simulink model "ETMX"  (R2017b)
settings: Solver=VariableStepAuto  StartTime=0.0  StopTime=10.0  RelTol=1e-3
undefined symbols (not defined in the file): sys1
settings Model: Creator=ayaka  LastModifiedBy=ayaka

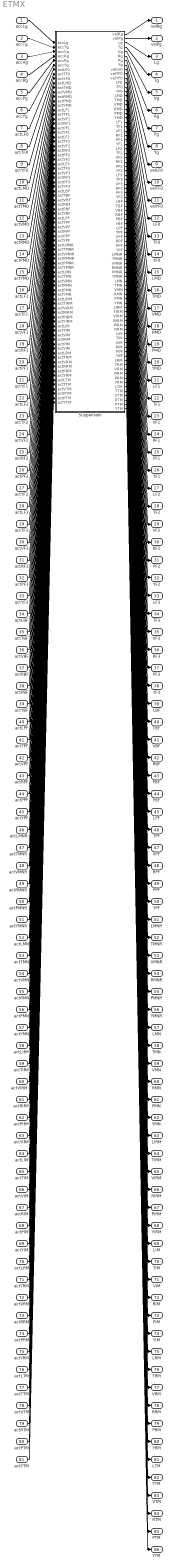
== system ETMX ==
  accLg : Inport
  accTg : Inport  Port=2
  accVg : Inport  Port=3
  accRg : Inport  Port=4
  accPg : Inport  Port=5
  accYg : Inport  Port=6
  actLF0 : Inport  Port=7
  actTF0 : Inport  Port=8
  actYF0 : Inport  Port=9
  actLMD : Inport  Port=10
  actTMD : Inport  Port=11
  actVMD : Inport  Port=12
  actRMD : Inport  Port=13
  actPMD : Inport  Port=14
  actYMD : Inport  Port=15
  actLF1 : Inport  Port=16
  actTF1 : Inport  Port=17
  actVF1 : Inport  Port=18
  actRF1 : Inport  Port=19
  actPF1 : Inport  Port=20
  actYF1 : Inport  Port=21
  actLF2 : Inport  Port=22
  actTF2 : Inport  Port=23
  actVF2 : Inport  Port=24
  actRF2 : Inport  Port=25
  actPF2 : Inport  Port=26
  actYF2 : Inport  Port=27
  actLF3 : Inport  Port=28
  actTF3 : Inport  Port=29
  actVF3 : Inport  Port=30
  actRF3 : Inport  Port=31
  actPF3 : Inport  Port=32
  actYF3 : Inport  Port=33
  actLBF : Inport  Port=34
  actTBF : Inport  Port=35
  actVBF : Inport  Port=36
  actRBF : Inport  Port=37
  actPBF : Inport  Port=38
  actYBF : Inport  Port=39
  actLPF : Inport  Port=40
  actTPF : Inport  Port=41
  actVPF : Inport  Port=42
  actRPF : Inport  Port=43
  actPPF : Inport  Port=44
  actYPF : Inport  Port=45
  actLMNR : Inport  Port=46
  actTMNR : Inport  Port=47
  actVMNR : Inport  Port=48
  actRMNR : Inport  Port=49
  actPMNR : Inport  Port=50
  actYMNR : Inport  Port=51
  actLMN : Inport  Port=52
  actTMN : Inport  Port=53
  actVMN : Inport  Port=54
  actRMN : Inport  Port=55
  actPMN : Inport  Port=56
  actYMN : Inport  Port=57
  actLIRM : Inport  Port=58
  actTIRM : Inport  Port=59
  actVIRM : Inport  Port=60
  actRIRM : Inport  Port=61
  actPIRM : Inport  Port=62
  actYIRM : Inport  Port=63
  actLIM : Inport  Port=64
  actTIM : Inport  Port=65
  actVIM : Inport  Port=66
  actRIM : Inport  Port=67
  actPIM : Inport  Port=68
  actYIM : Inport  Port=69
  actLRM : Inport  Port=70
  actTRM : Inport  Port=71
  actVRM : Inport  Port=72
  actRRM : Inport  Port=73
  actPRM : Inport  Port=74
  actYRM : Inport  Port=75
  actLTM : Inport  Port=76
  actTTM : Inport  Port=77
  actVTM : Inport  Port=78
  actRTM : Inport  Port=79
  actPTM : Inport  Port=80
  actYTM : Inport  Port=81
  Suspension : Subsystem
  velRg : Outport
  velPg : Outport  Port=2
  Lg : Outport  Port=3
  Tg : Outport  Port=4
  Vg : Outport  Port=5
  Rg : Outport  Port=6
  Pg : Outport  Port=7
  Yg : Outport  Port=8
  velLF0 : Outport  Port=9
  velTF0 : Outport  Port=10
  velYF0 : Outport  Port=11
  LF0 : Outport  Port=12
  TF0 : Outport  Port=13
  YF0 : Outport  Port=14
  LMD : Outport  Port=15
  TMD : Outport  Port=16
  VMD : Outport  Port=17
  RMD : Outport  Port=18
  PMD : Outport  Port=19
  YMD : Outport  Port=20
  LF1 : Outport  Port=21
  TF1 : Outport  Port=22
  VF1 : Outport  Port=23
  RF1 : Outport  Port=24
  PF1 : Outport  Port=25
  YF1 : Outport  Port=26
  LF2 : Outport  Port=27
  TF2 : Outport  Port=28
  VF2 : Outport  Port=29
  RF2 : Outport  Port=30
  PF2 : Outport  Port=31
  YF2 : Outport  Port=32
  LF3 : Outport  Port=33
  TF3 : Outport  Port=34
  VF3 : Outport  Port=35
  RF3 : Outport  Port=36
  PF3 : Outport  Port=37
  YF3 : Outport  Port=38
  LBF : Outport  Port=39
  TBF : Outport  Port=40
  VBF : Outport  Port=41
  RBF : Outport  Port=42
  PBF : Outport  Port=43
  YBF : Outport  Port=44
  LPF : Outport  Port=45
  TPF : Outport  Port=46
  VPF : Outport  Port=47
  RPF : Outport  Port=48
  PPF : Outport  Port=49
  YPF : Outport  Port=50
  LMNR : Outport  Port=51
  TMNR : Outport  Port=52
  VMNR : Outport  Port=53
  RMNR : Outport  Port=54
  PMNR : Outport  Port=55
  YMNR : Outport  Port=56
  LMN : Outport  Port=57
  TMN : Outport  Port=58
  VMN : Outport  Port=59
  RMN : Outport  Port=60
  PMN : Outport  Port=61
  YMN : Outport  Port=62
  LIRM : Outport  Port=63
  TIRM : Outport  Port=64
  VIRM : Outport  Port=65
  RIRM : Outport  Port=66
  PIRM : Outport  Port=67
  YIRM : Outport  Port=68
  LIM : Outport  Port=69
  TIM : Outport  Port=70
  VIM : Outport  Port=71
  RIM : Outport  Port=72
  PIM : Outport  Port=73
  YIM : Outport  Port=74
  LRM : Outport  Port=75
  TRM : Outport  Port=76
  VRM : Outport  Port=77
  RRM : Outport  Port=78
  PRM : Outport  Port=79
  YRM : Outport  Port=80
  LTM : Outport  Port=81
  TTM : Outport  Port=82
  VTM : Outport  Port=83
  RTM : Outport  Port=84
  PTM : Outport  Port=85
  YTM : Outport  Port=86
  wires:
  accLg/1 -> Suspension/1(accLg)
  accTg/1 -> Suspension/2(accTg)
  accVg/1 -> Suspension/3(accVg)
  accRg/1 -> Suspension/4(accRg)
  accPg/1 -> Suspension/5(accPg)
  accYg/1 -> Suspension/6(accYg)
  actLF0/1 -> Suspension/7(actLF0)
  actTF0/1 -> Suspension/8(actTF0)
  actYF0/1 -> Suspension/9(actYF0)
  actLMD/1 -> Suspension/10(actLMD)
  actTMD/1 -> Suspension/11(actTMD)
  actVMD/1 -> Suspension/12(actVMD)
  actRMD/1 -> Suspension/13(actRMD)
  actPMD/1 -> Suspension/14(actPMD)
  actYMD/1 -> Suspension/15(actYMD)
  actLF1/1 -> Suspension/16(actLF1)
  actTF1/1 -> Suspension/17(actTF1)
  actVF1/1 -> Suspension/18(actVF1)
  actRF1/1 -> Suspension/19(actRF1)
  actPF1/1 -> Suspension/20(actPF1)
  actYF1/1 -> Suspension/21(actYF1)
  actLF2/1 -> Suspension/22(actLF2)
  actTF2/1 -> Suspension/23(actTF2)
  actVF2/1 -> Suspension/24(actVF2)
  actRF2/1 -> Suspension/25(actRF2)
  actPF2/1 -> Suspension/26(actPF2)
  actYF2/1 -> Suspension/27(actYF2)
  actLF3/1 -> Suspension/28(actLF3)
  actTF3/1 -> Suspension/29(actTF3)
  actVF3/1 -> Suspension/30(actVF3)
  actRF3/1 -> Suspension/31(actRF3)
  actPF3/1 -> Suspension/32(actPF3)
  actYF3/1 -> Suspension/33(actYF3)
  actLBF/1 -> Suspension/34(actLBF)
  actTBF/1 -> Suspension/35(actTBF)
  actVBF/1 -> Suspension/36(actVBF)
  actRBF/1 -> Suspension/37(actRBF)
  actPBF/1 -> Suspension/38(actPBF)
  actYBF/1 -> Suspension/39(actYBF)
  actLPF/1 -> Suspension/40(actLPF)
  actTPF/1 -> Suspension/41(actTPF)
  actVPF/1 -> Suspension/42(actVPF)
  actRPF/1 -> Suspension/43(actRPF)
  actPPF/1 -> Suspension/44(actPPF)
  actYPF/1 -> Suspension/45(actYPF)
  actLMNR/1 -> Suspension/46(actLMNR)
  actTMNR/1 -> Suspension/47(actTMNR)
  actVMNR/1 -> Suspension/48(actVMNR)
  actRMNR/1 -> Suspension/49(actRMNR)
  actPMNR/1 -> Suspension/50(actPMNR)
  actYMNR/1 -> Suspension/51(actYMNR)
  actLMN/1 -> Suspension/52(actLMN)
  actTMN/1 -> Suspension/53(actTMN)
  actVMN/1 -> Suspension/54(actVMN)
  actRMN/1 -> Suspension/55(actRMN)
  actPMN/1 -> Suspension/56(actPMN)
  actYMN/1 -> Suspension/57(actYMN)
  actLIRM/1 -> Suspension/58(actLIRM)
  actTIRM/1 -> Suspension/59(actTIRM)
  actVIRM/1 -> Suspension/60(actVIRM)
  actRIRM/1 -> Suspension/61(actRIRM)
  actPIRM/1 -> Suspension/62(actPIRM)
  actYIRM/1 -> Suspension/63(actYIRM)
  actLIM/1 -> Suspension/64(actLIM)
  actTIM/1 -> Suspension/65(actTIM)
  actVIM/1 -> Suspension/66(actVIM)
  actRIM/1 -> Suspension/67(actRIM)
  actPIM/1 -> Suspension/68(actPIM)
  actYIM/1 -> Suspension/69(actYIM)
  actLRM/1 -> Suspension/70(actLRM)
  actTRM/1 -> Suspension/71(actTRM)
  actVRM/1 -> Suspension/72(actVRM)
  actRRM/1 -> Suspension/73(actRRM)
  actPRM/1 -> Suspension/74(actPRM)
  actYRM/1 -> Suspension/75(actYRM)
  actLTM/1 -> Suspension/76(actLTM)
  actTTM/1 -> Suspension/77(actTTM)
  actVTM/1 -> Suspension/78(actVTM)
  actRTM/1 -> Suspension/79(actRTM)
  actPTM/1 -> Suspension/80(actPTM)
  actYTM/1 -> Suspension/81(actYTM)
  Suspension/1(velRg) -> velRg/1
  Suspension/2(velPg) -> velPg/1
  Suspension/3(Lg) -> Lg/1
  Suspension/4(Tg) -> Tg/1
  Suspension/5(Vg) -> Vg/1
  Suspension/6(Rg) -> Rg/1
  Suspension/7(Pg) -> Pg/1
  Suspension/8(Yg) -> Yg/1
  Suspension/9(velLF0) -> velLF0/1
  Suspension/10(velTF0) -> velTF0/1
  Suspension/11(velYF0) -> velYF0/1
  Suspension/12(LF0) -> LF0/1
  Suspension/13(TF0) -> TF0/1
  Suspension/14(YF0) -> YF0/1
  Suspension/15(LMD) -> LMD/1
  Suspension/16(TMD) -> TMD/1
  Suspension/17(VMD) -> VMD/1
  Suspension/18(RMD) -> RMD/1
  Suspension/19(PMD) -> PMD/1
  Suspension/20(YMD) -> YMD/1
  Suspension/21(LF1) -> LF1/1
  Suspension/22(TF1) -> TF1/1
  Suspension/23(VF1) -> VF1/1
  Suspension/24(RF1) -> RF1/1
  Suspension/25(PF1) -> PF1/1
  Suspension/26(YF1) -> YF1/1
  Suspension/27(LF2) -> LF2/1
  Suspension/28(TF2) -> TF2/1
  Suspension/29(VF2) -> VF2/1
  Suspension/30(RF2) -> RF2/1
  Suspension/31(PF2) -> PF2/1
  Suspension/32(YF2) -> YF2/1
  Suspension/33(LF3) -> LF3/1
  Suspension/34(TF3) -> TF3/1
  Suspension/35(VF3) -> VF3/1
  Suspension/36(RF3) -> RF3/1
  Suspension/37(PF3) -> PF3/1
  Suspension/38(YF3) -> YF3/1
  Suspension/39(LBF) -> LBF/1
  Suspension/40(TBF) -> TBF/1
  Suspension/41(VBF) -> VBF/1
  Suspension/42(RBF) -> RBF/1
  Suspension/43(PBF) -> PBF/1
  Suspension/44(YBF) -> YBF/1
  Suspension/45(LPF) -> LPF/1
  Suspension/46(TPF) -> TPF/1
  Suspension/47(VPF) -> VPF/1
  Suspension/48(RPF) -> RPF/1
  Suspension/49(PPF) -> PPF/1
  Suspension/50(YPF) -> YPF/1
  Suspension/51(LMNR) -> LMNR/1
  Suspension/52(TMNR) -> TMNR/1
  Suspension/53(VMNR) -> VMNR/1
  Suspension/54(RMNR) -> RMNR/1
  Suspension/55(PMNR) -> PMNR/1
  Suspension/56(YMNR) -> YMNR/1
  Suspension/57(LMN) -> LMN/1
  Suspension/58(TMN) -> TMN/1
  Suspension/59(VMN) -> VMN/1
  Suspension/60(RMN) -> RMN/1
  Suspension/61(PMN) -> PMN/1
  Suspension/62(YMN) -> YMN/1
  Suspension/63(LIRM) -> LIRM/1
  Suspension/64(TIRM) -> TIRM/1
  Suspension/65(VIRM) -> VIRM/1
  Suspension/66(RIRM) -> RIRM/1
  Suspension/67(PIRM) -> PIRM/1
  Suspension/68(YIRM) -> YIRM/1
  Suspension/69(LIM) -> LIM/1
  Suspension/70(TIM) -> TIM/1
  Suspension/71(VIM) -> VIM/1
  Suspension/72(RIM) -> RIM/1
  Suspension/73(PIM) -> PIM/1
  Suspension/74(YIM) -> YIM/1
  Suspension/75(LRM) -> LRM/1
  Suspension/76(TRM) -> TRM/1
  Suspension/77(VRM) -> VRM/1
  Suspension/78(RRM) -> RRM/1
  Suspension/79(PRM) -> PRM/1
  Suspension/80(YRM) -> YRM/1
  Suspension/81(LTM) -> LTM/1
  Suspension/82(TTM) -> TTM/1
  Suspension/83(VTM) -> VTM/1
  Suspension/84(RTM) -> RTM/1
  Suspension/85(PTM) -> PTM/1
  Suspension/86(YTM) -> YTM/1

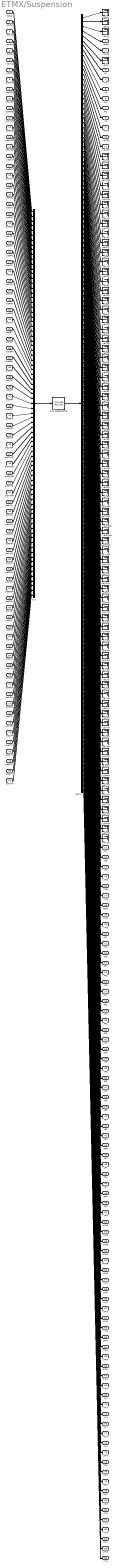
== system ETMX/Suspension ==
  accLg : Inport
  accTg : Inport  Port=2
  accVg : Inport  Port=3
  accRg : Inport  Port=4
  accPg : Inport  Port=5
  accYg : Inport  Port=6
  actLF0 : Inport  Port=7
  actTF0 : Inport  Port=8
  actYF0 : Inport  Port=9
  actLMD : Inport  Port=10
  actTMD : Inport  Port=11
  actVMD : Inport  Port=12
  actRMD : Inport  Port=13
  actPMD : Inport  Port=14
  actYMD : Inport  Port=15
  actLF1 : Inport  Port=16
  actTF1 : Inport  Port=17
  actVF1 : Inport  Port=18
  actRF1 : Inport  Port=19
  actPF1 : Inport  Port=20
  actYF1 : Inport  Port=21
  actLF2 : Inport  Port=22
  actTF2 : Inport  Port=23
  actVF2 : Inport  Port=24
  actRF2 : Inport  Port=25
  actPF2 : Inport  Port=26
  actYF2 : Inport  Port=27
  actLF3 : Inport  Port=28
  actTF3 : Inport  Port=29
  actVF3 : Inport  Port=30
  actRF3 : Inport  Port=31
  actPF3 : Inport  Port=32
  actYF3 : Inport  Port=33
  actLBF : Inport  Port=34
  actTBF : Inport  Port=35
  actVBF : Inport  Port=36
  actRBF : Inport  Port=37
  actPBF : Inport  Port=38
  actYBF : Inport  Port=39
  actLPF : Inport  Port=40
  actTPF : Inport  Port=41
  actVPF : Inport  Port=42
  actRPF : Inport  Port=43
  actPPF : Inport  Port=44
  actYPF : Inport  Port=45
  actLMNR : Inport  Port=46
  actTMNR : Inport  Port=47
  actVMNR : Inport  Port=48
  actRMNR : Inport  Port=49
  actPMNR : Inport  Port=50
  actYMNR : Inport  Port=51
  actLMN : Inport  Port=52
  actTMN : Inport  Port=53
  actVMN : Inport  Port=54
  actRMN : Inport  Port=55
  actPMN : Inport  Port=56
  actYMN : Inport  Port=57
  actLIRM : Inport  Port=58
  actTIRM : Inport  Port=59
  actVIRM : Inport  Port=60
  actRIRM : Inport  Port=61
  actPIRM : Inport  Port=62
  actYIRM : Inport  Port=63
  actLIM : Inport  Port=64
  actTIM : Inport  Port=65
  actVIM : Inport  Port=66
  actRIM : Inport  Port=67
  actPIM : Inport  Port=68
  actYIM : Inport  Port=69
  actLRM : Inport  Port=70
  actTRM : Inport  Port=71
  actVRM : Inport  Port=72
  actRRM : Inport  Port=73
  actPRM : Inport  Port=74
  actYRM : Inport  Port=75
  actLTM : Inport  Port=76
  actTTM : Inport  Port=77
  actVTM : Inport  Port=78
  actRTM : Inport  Port=79
  actPTM : Inport  Port=80
  actYTM : Inport  Port=81
  SAS State-Space : StateSpace  A=sys1.A  B=sys1.B  C=sys1.C  D=sys1.D  InitialCondition=0  ContinuousStateAttributes='SUS_SS_MODEL'
  demux : Demux  Outputs=162
  mux : Mux  Inputs=81
  velLBF : Terminator
  velLF1 : Terminator
  velLF2 : Terminator
  velLF3 : Terminator
  velLIM : Terminator
  velLIRM : Terminator
  velLMD : Terminator
  velLMN : Terminator
  velLMNR : Terminator
  velLPF : Terminator
  velLRM : Terminator
  velLTM : Terminator
  velLg : Terminator
  velPBF : Terminator
  velPF1 : Terminator
  velPF2 : Terminator
  velPF3 : Terminator
  velPIM : Terminator
  velPIRM : Terminator
  velPMD : Terminator
  velPMN : Terminator
  velPMNR : Terminator
  velPPF : Terminator
  velPRM : Terminator
  velPTM : Terminator
  velRBF : Terminator
  velRF1 : Terminator
  velRF2 : Terminator
  velRF3 : Terminator
  velRIM : Terminator
  velRIRM : Terminator
  velRMD : Terminator
  velRMN : Terminator
  velRMNR : Terminator
  velRPF : Terminator
  velRRM : Terminator
  velRTM : Terminator
  velTBF : Terminator
  velTF1 : Terminator
  velTF2 : Terminator
  velTF3 : Terminator
  velTIM : Terminator
  velTIRM : Terminator
  velTMD : Terminator
  velTMN : Terminator
  velTMNR : Terminator
  velTPF : Terminator
  velTRM : Terminator
  velTTM : Terminator
  velTg : Terminator
  velVBF : Terminator
  velVF1 : Terminator
  velVF2 : Terminator
  velVF3 : Terminator
  velVIM : Terminator
  velVIRM : Terminator
  velVMD : Terminator
  velVMN : Terminator
  velVMNR : Terminator
  velVPF : Terminator
  velVRM : Terminator
  velVTM : Terminator
  velVg : Terminator
  velYBF : Terminator
  velYF1 : Terminator
  velYF2 : Terminator
  velYF3 : Terminator
  velYIM : Terminator
  velYIRM : Terminator
  velYMD : Terminator
  velYMN : Terminator
  velYMNR : Terminator
  velYPF : Terminator
  velYRM : Terminator
  velYTM : Terminator
  velYg : Terminator
  velRg : Outport
  velPg : Outport  Port=2
  Lg : Outport  Port=3
  Tg : Outport  Port=4
  Vg : Outport  Port=5
  Rg : Outport  Port=6
  Pg : Outport  Port=7
  Yg : Outport  Port=8
  velLF0 : Outport  Port=9
  velTF0 : Outport  Port=10
  velYF0 : Outport  Port=11
  LF0 : Outport  Port=12
  TF0 : Outport  Port=13
  YF0 : Outport  Port=14
  LMD : Outport  Port=15
  TMD : Outport  Port=16
  VMD : Outport  Port=17
  RMD : Outport  Port=18
  PMD : Outport  Port=19
  YMD : Outport  Port=20
  LF1 : Outport  Port=21
  TF1 : Outport  Port=22
  VF1 : Outport  Port=23
  RF1 : Outport  Port=24
  PF1 : Outport  Port=25
  YF1 : Outport  Port=26
  LF2 : Outport  Port=27
  TF2 : Outport  Port=28
  VF2 : Outport  Port=29
  RF2 : Outport  Port=30
  PF2 : Outport  Port=31
  YF2 : Outport  Port=32
  LF3 : Outport  Port=33
  TF3 : Outport  Port=34
  VF3 : Outport  Port=35
  RF3 : Outport  Port=36
  PF3 : Outport  Port=37
  YF3 : Outport  Port=38
  LBF : Outport  Port=39
  TBF : Outport  Port=40
  VBF : Outport  Port=41
  RBF : Outport  Port=42
  PBF : Outport  Port=43
  YBF : Outport  Port=44
  LPF : Outport  Port=45
  TPF : Outport  Port=46
  VPF : Outport  Port=47
  RPF : Outport  Port=48
  PPF : Outport  Port=49
  YPF : Outport  Port=50
  LMNR : Outport  Port=51
  TMNR : Outport  Port=52
  VMNR : Outport  Port=53
  RMNR : Outport  Port=54
  PMNR : Outport  Port=55
  YMNR : Outport  Port=56
  LMN : Outport  Port=57
  TMN : Outport  Port=58
  VMN : Outport  Port=59
  RMN : Outport  Port=60
  PMN : Outport  Port=61
  YMN : Outport  Port=62
  LIRM : Outport  Port=63
  TIRM : Outport  Port=64
  VIRM : Outport  Port=65
  RIRM : Outport  Port=66
  PIRM : Outport  Port=67
  YIRM : Outport  Port=68
  LIM : Outport  Port=69
  TIM : Outport  Port=70
  VIM : Outport  Port=71
  RIM : Outport  Port=72
  PIM : Outport  Port=73
  YIM : Outport  Port=74
  LRM : Outport  Port=75
  TRM : Outport  Port=76
  VRM : Outport  Port=77
  RRM : Outport  Port=78
  PRM : Outport  Port=79
  YRM : Outport  Port=80
  LTM : Outport  Port=81
  TTM : Outport  Port=82
  VTM : Outport  Port=83
  RTM : Outport  Port=84
  PTM : Outport  Port=85
  YTM : Outport  Port=86
  wires:
  mux/1 -> SAS State-Space/1
  SAS State-Space/1 -> demux/1
  accLg/1 -> mux/1
  accTg/1 -> mux/2
  accVg/1 -> mux/3
  accRg/1 -> mux/4
  accPg/1 -> mux/5
  accYg/1 -> mux/6
  actLF0/1 -> mux/7
  actTF0/1 -> mux/8
  actYF0/1 -> mux/9
  actLMD/1 -> mux/10
  actTMD/1 -> mux/11
  actVMD/1 -> mux/12
  actRMD/1 -> mux/13
  actPMD/1 -> mux/14
  actYMD/1 -> mux/15
  actLF1/1 -> mux/16
  actTF1/1 -> mux/17
  actVF1/1 -> mux/18
  actRF1/1 -> mux/19
  actPF1/1 -> mux/20
  actYF1/1 -> mux/21
  actLF2/1 -> mux/22
  actTF2/1 -> mux/23
  actVF2/1 -> mux/24
  actRF2/1 -> mux/25
  actPF2/1 -> mux/26
  actYF2/1 -> mux/27
  actLF3/1 -> mux/28
  actTF3/1 -> mux/29
  actVF3/1 -> mux/30
  actRF3/1 -> mux/31
  actPF3/1 -> mux/32
  actYF3/1 -> mux/33
  actLBF/1 -> mux/34
  actTBF/1 -> mux/35
  actVBF/1 -> mux/36
  actRBF/1 -> mux/37
  actPBF/1 -> mux/38
  actYBF/1 -> mux/39
  actLPF/1 -> mux/40
  actTPF/1 -> mux/41
  actVPF/1 -> mux/42
  actRPF/1 -> mux/43
  actPPF/1 -> mux/44
  actYPF/1 -> mux/45
  actLMNR/1 -> mux/46
  actTMNR/1 -> mux/47
  actVMNR/1 -> mux/48
  actRMNR/1 -> mux/49
  actPMNR/1 -> mux/50
  actYMNR/1 -> mux/51
  actLMN/1 -> mux/52
  actTMN/1 -> mux/53
  actVMN/1 -> mux/54
  actRMN/1 -> mux/55
  actPMN/1 -> mux/56
  actYMN/1 -> mux/57
  actLIRM/1 -> mux/58
  actTIRM/1 -> mux/59
  actVIRM/1 -> mux/60
  actRIRM/1 -> mux/61
  actPIRM/1 -> mux/62
  actYIRM/1 -> mux/63
  actLIM/1 -> mux/64
  actTIM/1 -> mux/65
  actVIM/1 -> mux/66
  actRIM/1 -> mux/67
  actPIM/1 -> mux/68
  actYIM/1 -> mux/69
  actLRM/1 -> mux/70
  actTRM/1 -> mux/71
  actVRM/1 -> mux/72
  actRRM/1 -> mux/73
  actPRM/1 -> mux/74
  actYRM/1 -> mux/75
  actLTM/1 -> mux/76
  actTTM/1 -> mux/77
  actVTM/1 -> mux/78
  actRTM/1 -> mux/79
  actPTM/1 -> mux/80
  actYTM/1 -> mux/81
  demux/1 -> velLg/1
  demux/2 -> velTg/1
  demux/3 -> velVg/1
  demux/4 -> velRg/1
  demux/5 -> velPg/1
  demux/6 -> velYg/1
  demux/7 -> Lg/1
  demux/8 -> Tg/1
  demux/9 -> Vg/1
  demux/10 -> Rg/1
  demux/11 -> Pg/1
  demux/12 -> Yg/1
  demux/13 -> velLF0/1
  demux/14 -> velTF0/1
  demux/15 -> velYF0/1
  demux/16 -> velLMD/1
  demux/17 -> velTMD/1
  demux/18 -> velVMD/1
  demux/19 -> velRMD/1
  demux/20 -> velPMD/1
  demux/21 -> velYMD/1
  demux/22 -> velLF1/1
  demux/23 -> velTF1/1
  demux/24 -> velVF1/1
  demux/25 -> velRF1/1
  demux/26 -> velPF1/1
  demux/27 -> velYF1/1
  demux/28 -> velLF2/1
  demux/29 -> velTF2/1
  demux/30 -> velVF2/1
  demux/31 -> velRF2/1
  demux/32 -> velPF2/1
  demux/33 -> velYF2/1
  demux/34 -> velLF3/1
  demux/35 -> velTF3/1
  demux/36 -> velVF3/1
  demux/37 -> velRF3/1
  demux/38 -> velPF3/1
  demux/39 -> velYF3/1
  demux/40 -> velLBF/1
  demux/41 -> velTBF/1
  demux/42 -> velVBF/1
  demux/43 -> velRBF/1
  demux/44 -> velPBF/1
  demux/45 -> velYBF/1
  demux/46 -> velLPF/1
  demux/47 -> velTPF/1
  demux/48 -> velVPF/1
  demux/49 -> velRPF/1
  demux/50 -> velPPF/1
  demux/51 -> velYPF/1
  demux/52 -> velLMNR/1
  demux/53 -> velTMNR/1
  demux/54 -> velVMNR/1
  demux/55 -> velRMNR/1
  demux/56 -> velPMNR/1
  demux/57 -> velYMNR/1
  demux/58 -> velLMN/1
  demux/59 -> velTMN/1
  demux/60 -> velVMN/1
  demux/61 -> velRMN/1
  demux/62 -> velPMN/1
  demux/63 -> velYMN/1
  demux/64 -> velLIRM/1
  demux/65 -> velTIRM/1
  demux/66 -> velVIRM/1
  demux/67 -> velRIRM/1
  demux/68 -> velPIRM/1
  demux/69 -> velYIRM/1
  demux/70 -> velLIM/1
  demux/71 -> velTIM/1
  demux/72 -> velVIM/1
  demux/73 -> velRIM/1
  demux/74 -> velPIM/1
  demux/75 -> velYIM/1
  demux/76 -> velLRM/1
  demux/77 -> velTRM/1
  demux/78 -> velVRM/1
  demux/79 -> velRRM/1
  demux/80 -> velPRM/1
  demux/81 -> velYRM/1
  demux/82 -> velLTM/1
  demux/83 -> velTTM/1
  demux/84 -> velVTM/1
  demux/85 -> velRTM/1
  demux/86 -> velPTM/1
  demux/87 -> velYTM/1
  demux/88 -> LF0/1
  demux/89 -> TF0/1
  demux/90 -> YF0/1
  demux/91 -> LMD/1
  demux/92 -> TMD/1
  demux/93 -> VMD/1
  demux/94 -> RMD/1
  demux/95 -> PMD/1
  demux/96 -> YMD/1
  demux/97 -> LF1/1
  demux/98 -> TF1/1
  demux/99 -> VF1/1
  demux/100 -> RF1/1
  demux/101 -> PF1/1
  demux/102 -> YF1/1
  demux/103 -> LF2/1
  demux/104 -> TF2/1
  demux/105 -> VF2/1
  demux/106 -> RF2/1
  demux/107 -> PF2/1
  demux/108 -> YF2/1
  demux/109 -> LF3/1
  demux/110 -> TF3/1
  demux/111 -> VF3/1
  demux/112 -> RF3/1
  demux/113 -> PF3/1
  demux/114 -> YF3/1
  demux/115 -> LBF/1
  demux/116 -> TBF/1
  demux/117 -> VBF/1
  demux/118 -> RBF/1
  demux/119 -> PBF/1
  demux/120 -> YBF/1
  demux/121 -> LPF/1
  demux/122 -> TPF/1
  demux/123 -> VPF/1
  demux/124 -> RPF/1
  demux/125 -> PPF/1
  demux/126 -> YPF/1
  demux/127 -> LMNR/1
  demux/128 -> TMNR/1
  demux/129 -> VMNR/1
  demux/130 -> RMNR/1
  demux/131 -> PMNR/1
  demux/132 -> YMNR/1
  demux/133 -> LMN/1
  demux/134 -> TMN/1
  demux/135 -> VMN/1
  demux/136 -> RMN/1
  demux/137 -> PMN/1
  demux/138 -> YMN/1
  demux/139 -> LIRM/1
  demux/140 -> TIRM/1
  demux/141 -> VIRM/1
  demux/142 -> RIRM/1
  demux/143 -> PIRM/1
  demux/144 -> YIRM/1
  demux/145 -> LIM/1
  demux/146 -> TIM/1
  demux/147 -> VIM/1
  demux/148 -> RIM/1
  demux/149 -> PIM/1
  demux/150 -> YIM/1
  demux/151 -> LRM/1
  demux/152 -> TRM/1
  demux/153 -> VRM/1
  demux/154 -> RRM/1
  demux/155 -> PRM/1
  demux/156 -> YRM/1
  demux/157 -> LTM/1
  demux/158 -> TTM/1
  demux/159 -> VTM/1
  demux/160 -> RTM/1
  demux/161 -> PTM/1
  demux/162 -> YTM/1
